simulink model "CompressorDesign"  (R2016b)
settings: Solver=FixedStepDiscrete  StartTime=0.0  StopTime=inf  RelTol=1e-3
libraries: dspvision x2, dspsnks4 x1, dspmathops x1
settings Model: Creator=michaelseaberg  LastModifiedBy=michaelseaberg
settings SolverCC: AutoInsertRateTranBlk=on
settings DataIOCC: LimitDataPoints=on  SaveOutput=off  SignalLogging=off  SaveTime=off
settings OptimizationCC: LifeSpan=inf
settings DebuggingCC: AlgebraicLoopMsg=error  SingleTaskRateTransMsg=error  AllowSymbolicDim=off  SFUnexpectedBacktrackingDiag=warning  SFNoUnconditionalDefaultTransitionDiag=warning  SFExecutionAtInitializationDiag=none
settings GRTTargetCC: TargetLangStandard=C89/C90 (ANSI)  GeneratePreprocessorConditionals=Disable all
settings ConfigComp: CovMetricSettings=dw  CovHtmlReporting=on  CovSaveCumulativeToWorkspaceVar=on  CovSaveSingleToWorkspaceVar=on  CovExternalEMLEnable=off  CovSFcnEnable=off

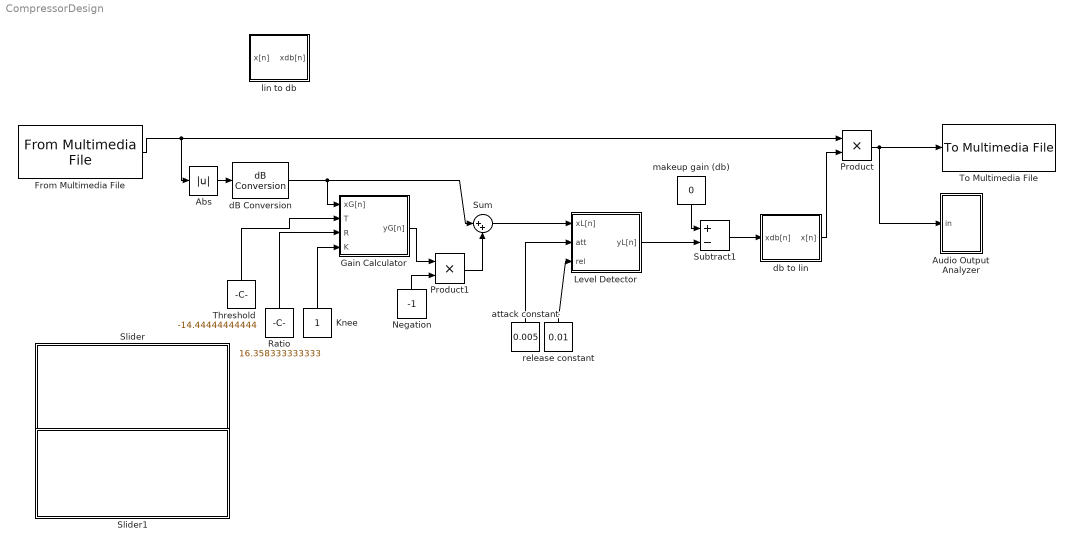
== system CompressorDesign ==
  Abs : Abs
  "Audio Output Analyzer " : Subsystem
  From Multimedia File : dspvision/From Multimedia File  inputFilename=/Users/michaelseaberg/Music/Logic/str final project/Audio Files/Vocal.wav  loop=on  numPlays=inf  outputStreams=Audio only  videoDataType=single  audioDataType=double  inheritSampleTime=on  userDefinedSampleTime=1/30  noAudioOutput=off  isIntensityVideo=off  fourcc=RGB  colorVideoFormat=Separate color signals  outputEOF=off  dataOrg=Column-major  audioFrameSize=1024  computeAudioFrameSize=off  outSamplingMode=Sample based
  Gain Calculator : Subsystem
  Knee : Constant
  Level Detector : Subsystem
  Negation : Constant  Value=-1
  Product : Product
  Product1 : Product
  Ratio : Constant  Value=16.358333333333
  Slider : Subsystem  DialogController=hmiCreateDDGDialog  IsWebBlock=on  mask(MWDashboardBlock){webBlockId=81e3e5d4-3e7c-4834-98be-97a71d78d1c4, webBlockType=slider, ShowInLibBrowser=on, ShowInitialText=on, HMISrcModelName=CompressorDesign}
      mask prompts: webBlockId "WebBlock Id"; webBlockType "WebBlock Type"; HMISrcModelName "Source Model"
      mask help: SimulinkHMI:dialogs:SliderDialogDesc
      mask Help: helpview([docroot '/mapfiles/simulink.map'], 'hmi_slider')
      mask Display:
      | if strcmp(get_param(bdroot(gcb),'BlockDiagramType'), 'library')
      |     image([(matlabroot) '/toolbox/simulink/hmi/icons/Slider.png']);
      | end
  Slider1 : Subsystem  DialogController=hmiCreateDDGDialog  IsWebBlock=on  mask(MWDashboardBlock){webBlockId=f4b37f63-6bae-476a-9e0a-544a33ca854d, webBlockType=slider, ShowInLibBrowser=on, ShowInitialText=on, HMISrcModelName=CompressorDesign}
      mask prompts: webBlockId "WebBlock Id"; webBlockType "WebBlock Type"; HMISrcModelName "Source Model"
      mask help: SimulinkHMI:dialogs:SliderDialogDesc
      mask Help: helpview([docroot '/mapfiles/simulink.map'], 'hmi_slider')
      mask Display:
      | if strcmp(get_param(bdroot(gcb),'BlockDiagramType'), 'library')
      |     image([(matlabroot) '/toolbox/simulink/hmi/icons/Slider.png']);
      | end
  Subtract1 : Sum  Inputs=+-
  Sum : Sum  Inputs=|++
  Threshold : Constant  Value=-14.44444444444
  To Multimedia File : dspvision/To Multimedia File  outputFilename=output.wav  streamSelection=Audio only  videoCompressor=None (uncompressed)  audioCompressor=None (uncompressed)  imagePorts=Separate color signals  fileType=WAV  audioDatatype=16-bit integer  fourcc=RGB  videoQuality=75  mj2000CompFactor=10
  attack constant : Constant  Value=0.005
  dB Conversion : dspmathops/dB Conversion  dBtype=dB  intype=Amplitude  R=1  fuzz=on
  "db to lin " : Subsystem
  "lin to db " : Subsystem
  "makeup gain (db) " : Constant  Value=0
  release constant : Constant  Value=0.01
  wires:
  "db to lin "/1(x[n]) -> Product/2
  From Multimedia File/1 -> Abs/1, Product/1
  Threshold/1 -> Gain Calculator/2("T ")
  Ratio/1 -> Gain Calculator/3("R ")
  Knee/1 -> Gain Calculator/4(K)
  Sum/1 -> Level Detector/1(xL[n])
  release constant/1 -> Level Detector/3(rel)
  attack constant/1 -> Level Detector/2("att ")
  Subtract1/1 -> "db to lin "/1(xdb[n])
  Level Detector/1(yL[n]) -> Subtract1/2
  "makeup gain (db) "/1 -> Subtract1/1
  Product/1 -> "Audio Output Analyzer "/1(in), To Multimedia File/1
  Abs/1 -> dB Conversion/1
  dB Conversion/1 -> Sum/1, Gain Calculator/1(xG[n])
  Gain Calculator/1(yG[n]) -> Product1/1
  Negation/1 -> Product1/2
  Product1/1 -> Sum/2

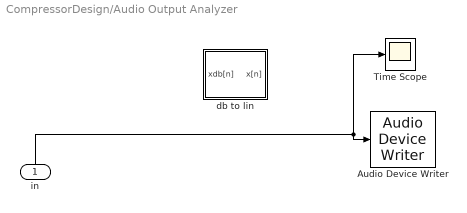
== system CompressorDesign/Audio Output Analyzer  ==
  in : Inport
  Audio Device Writer : dspsnks4/Audio Device Writer  Driver=CoreAudio  Device=Built-in Output  InheritSampleRate=on  SampleRate=44100  BitDepth=16-bit integer  BufferSize=4096  NumBuffers=10  DefaultOutputChannelMapping=on  OutputChannelMapping=1:2  OutputNumUnderrunSamples=off  DriverIdx=5  DeviceWarnFlag=''
  Time Scope : Scope
  "db to lin " : Subsystem
  wires:
  in/1 -> Audio Device Writer/1, Time Scope/1

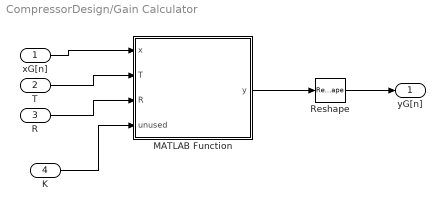
== system CompressorDesign/Gain Calculator ==
  xG[n] : Inport
  "T " : Inport  Port=2
  "R " : Inport  Port=3
  K : Inport  Port=4
  MATLAB Function : MATLAB Function  TreatAsAtomicUnit=on
  Reshape : Reshape  OutputDimensionality=Column vector (2-D)
  yG[n] : Outport
  wires:
  MATLAB Function/1(y) -> Reshape/1
  xG[n]/1 -> MATLAB Function/1(x)
  "T "/1 -> MATLAB Function/2(T)
  "R "/1 -> MATLAB Function/3(R)
  K/1 -> MATLAB Function/4(unused)
  Reshape/1 -> yG[n]/1

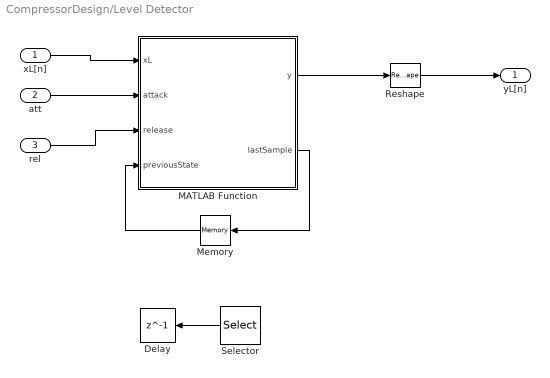
== system CompressorDesign/Level Detector ==
  xL[n] : Inport
  "att " : Inport  Port=2
  rel : Inport  Port=3
  Delay : Delay  DelayLength=1  InitialCondition=0
  MATLAB Function : MATLAB Function  TreatAsAtomicUnit=on
  Memory : Memory
  Reshape : Reshape  OutputDimensionality=Column vector (2-D)
  Selector : Selector  NumberOfDimensions=2  InputPortWidth=1024  IndexOptions=Index vector (dialog),Index vector (dialog)  Indices=1024,1  OutputSizes=1,1
  yL[n] : Outport
  wires:
  MATLAB Function/1(y) -> Reshape/1
  xL[n]/1 -> MATLAB Function/1(xL)
  "att "/1 -> MATLAB Function/2(attack)
  rel/1 -> MATLAB Function/3(release)
  Selector/1 -> Delay/1
  MATLAB Function/2(lastSample) -> Memory/1
  Memory/1 -> MATLAB Function/4(previousState)
  Reshape/1 -> yL[n]/1

== system CompressorDesign/Slider ==

== system CompressorDesign/Slider1 ==

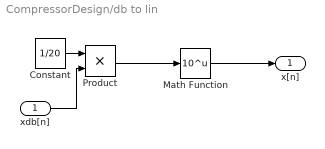
== system CompressorDesign/db to lin  ==
  xdb[n] : Inport
  Constant : Constant  Value=1/20
  Math Function : Math  Operator=10^u  SaturateOnIntegerOverflow=on
  Product : Product
  x[n] : Outport
  wires:
  Constant/1 -> Product/1
  xdb[n]/1 -> Product/2
  Product/1 -> Math Function/1
  Math Function/1 -> x[n]/1

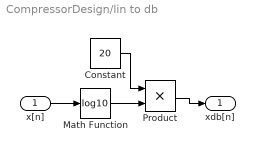
== system CompressorDesign/lin to db  ==
  x[n] : Inport
  Constant : Constant  Value=20
  Math Function : Math  Operator=log10  SaturateOnIntegerOverflow=on
  Product : Product
  xdb[n] : Outport
  wires:
  x[n]/1 -> Math Function/1
  Math Function/1 -> Product/2
  Product/1 -> xdb[n]/1
  Constant/1 -> Product/1

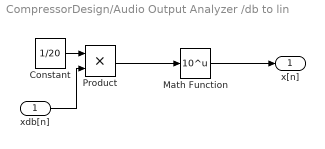
== system CompressorDesign/Audio Output Analyzer /db to lin  ==
  xdb[n] : Inport
  Constant : Constant  Value=1/20
  Math Function : Math  Operator=10^u  SaturateOnIntegerOverflow=on
  Product : Product
  x[n] : Outport
  wires:
  Constant/1 -> Product/1
  xdb[n]/1 -> Product/2
  Product/1 -> Math Function/1
  Math Function/1 -> x[n]/1

== matlab function CompressorDesign/Level Detector/MATLAB Function ==
  data: xL input; y output; attack input; release input; previousState input; lastSample output
function [y,lastSample] = levelDetector(xL,attack,release,previousState)

output = zeros(length(xL),1);
for n=1:length(xL)
    if xL(n) > previousState
        output(n,1) = attack.*previousState+(1-attack).*xL(n,1);
    else
        output(n,1) = release.*previousState+(1-release).*xL(n,1);
    end
    previousState = output(n,1);
end

lastSample = output(length(xL),1);
y = output;

== matlab function CompressorDesign/Gain Calculator/MATLAB Function ==
  data: x input; y output; T input; R input; unused input
function y = gainCalculator(x,T,R,~)
y = zeros(size(x));

for n=1:length(x)
    
    if x(n)<=T
        y(n,1) = x(n,1);
    else
        y(n,1) = T+(x(n,1)-T)./R;
    end
end
